simulink model "Linearization2"  (R2022a)
settings: Solver=VariableStepAuto  StartTime=0.0  StopTime=10.0  RelTol=1e-3
undefined symbols (not defined in the file): Aactuator, ac, AeroCoeff, ControlAllocation, DUmax, DUmin, EngineTable, F, fcs, ft, g, hground, IC, kg, LandingGear, Light, LPmethod, m, MIL, Mode_deflection_aileron, Mode_deflection_elevator, Mode_deflection_rudder, Mode_deflection_TVC_y, Mode_deflection_TVC_z, N, Ninv_2nozzle, Ninv_no_nozzle, PIController, s, Sensor, slug, state0, sysID_DAQ, sysID_OBES, Umax_2nozzle, Umax_no_nozzle, Umin_2nozzle, Umin_no_nozzle, WMM2020
libraries: aerolibconvert2 x19, slpidlib x6, simulink x6, sharedutil x4, aerolibatmos2 x3, aerolibwind2 x3, aerolibbdyn x3, aerolibgravity2 x2, sharedtransform x1
(part 1 of 9)
settings Model: Creator=user  LastModifiedBy=user
settings DataIOCC: ExternalInput=getinputstruct(op_trim1)  InitialState=getstatestruct(op_trim1)

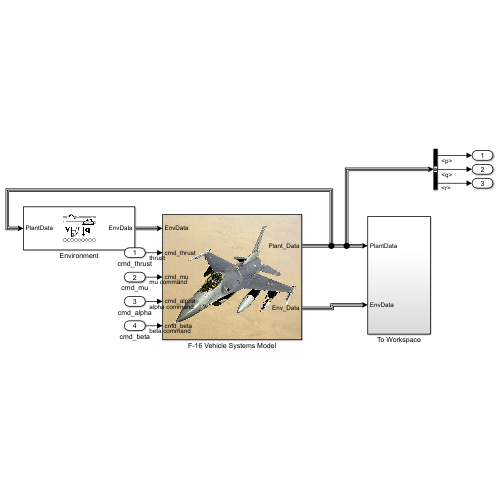
[thumbnail: Simulink's stored preview of the top-level diagram]
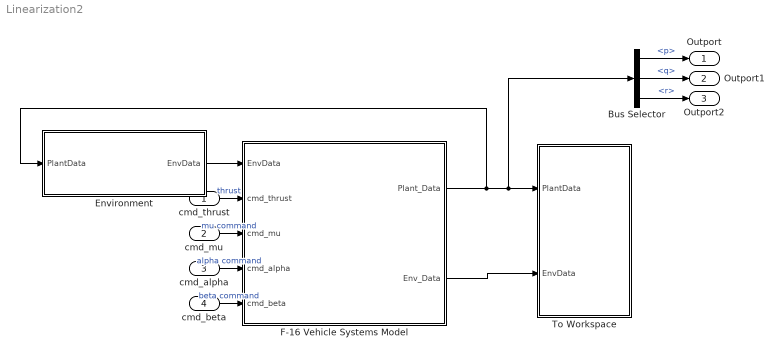
== system Linearization2 ==
  cmd_thrust : Inport
  cmd_mu : Inport  Port=2
  cmd_alpha : Inport  Port=3
  cmd_beta : Inport  Port=4
  Bus Selector : BusSelector  OutputSignals=p,q,r
  Environment : Subsystem
      mask Display:
      | image('aeroenvironment.bmp','center')
      | % 左側 "Icon transparency" 欄位已選擇 "Opaque with ports"，所以埠名稱會自動顯示，不用再宣告
      | % port_label('input',1,'PlantData')
      | % port_label('output',1,'EnvData')
  F-16 Vehicle Systems Model : Subsystem
      mask Display:
      | proj = currentProject;   % 返回一個專案物件proj 代表當前打開的Project專案
      | filepath = fullfile(proj.RootFolder,'\image\F-16_wikipedia.jpg');
      | image(filepath,'center');
      | % 左側 "Icon transparency" 欄位已選擇 "Opaque with ports"，所以埠名稱會自動顯示，不用再宣告
      | % port_label('input',1,'EnvData')
      | % port_label('output',1,'Plant_Data')
      | % port_label('output',2,'Env_Data')
  To Workspace : Subsystem
  Outport : Outport
  Outport1 : Outport  Port=2
  Outport2 : Outport  Port=3
  wires:
  F-16 Vehicle Systems Model/1(Plant_Data) -> Environment/1(PlantData), Bus Selector/1, To Workspace/1(PlantData)
  F-16 Vehicle Systems Model/2(Env_Data) -> To Workspace/2(EnvData)
  Environment/1(EnvData) -> F-16 Vehicle Systems Model/1(EnvData)
  cmd_thrust/1 -> F-16 Vehicle Systems Model/2(cmd_thrust)  "thrust"
  cmd_mu/1 -> F-16 Vehicle Systems Model/3(cmd_mu)  "mu command"
  cmd_alpha/1 -> F-16 Vehicle Systems Model/4(cmd_alpha)  "alpha command"
  cmd_beta/1 -> F-16 Vehicle Systems Model/5(cmd_beta)  "beta command"
  Bus Selector/1 -> Outport/1  "<p>"
  Bus Selector/2 -> Outport1/1  "<q>"
  Bus Selector/3 -> Outport2/1  "<r>"

== system Linearization2/Environment ==
  note: p, q, r
  note: u, v, w
  note: Wind Models
  note: Atmosphere Model
  note: Altitude must be less than 20000 m (approximately 65620 feet).
  note: 建模注意： EnvData Bus 內要指定公制/英制單位
  note: Magnetic Field
  note: Gravity Model
  note: TODO: 改用這個現成模塊...
      | 但NDI控制器內的重力g是用常數，將產生誤差...
  note: TODO: 改用這個現成模塊...
      | 參考MATLAB Help範例 Quadcopter Project
  note: TODO: 改用現成模塊，改成英制。
      | NDI控制器，不會產生誤差，因為可轉成C程式碼
  note: TODO: 參考MATLAB Help範例 HL-20
      | 將風速效應加到氣動力攻角、側滑角、qbar、Mach、V
  In Bus Element1 : Inport  PortName=PlantData  Element=altitude
  In Bus Element2 : Inport  PortName=PlantData  Element=altitude
  In Bus Element3 : Inport  PortName=PlantData  Element=Vt
  In Bus Element4 : Inport  PortName=PlantData  Element=Vt
  In Bus Element5 : Inport  PortName=PlantData  Element=Vt
  In Bus Element : Inport  PortName=PlantData  Element=DCM_be
  COESA Atmosphere Model : aerolibatmos2/COESA Atmosphere Model  Commented=on  units=English (Velocity in ft/s)  spec=1976 COESA-extended U.S. Standard Atmosphere  model=Profile  profile_var=High temperature  profile_percent=1%  profile_alt=5 km (16404 ft)  envelope_var=High temperature  envelope_percent=1%  action=Warning
  Density Conversion : aerolibconvert2/Density Conversion  IU=kg/m^3  OU=slug/ft^3
      settings: SourceProductBaseCode=AE
  Discrete Wind Gust Model : aerolibwind2/Discrete Wind Gust Model  Commented=on  units=English (Velocity in ft/s)  Gx=on  Gy=on  Gz=on  t_0=5  d_m=[120 120 80]  v_m=[3.5 3.5 3.0]
  Dryden Wind Turbulence Model (Continuous (+q +r)) : aerolibwind2/Dryden Wind Turbulence Model  (Continuous (+q -r))  Commented=on  units=English (Velocity in ft/s)  spec=MIL-F-8785C  model=Continuous Dryden (+q +r)  W20=15  Wdeg=0  TurbProb=10^-2 - Light  L_high=533.4  Wingspan=10  ts=0.1  Seed=[23341 23342 23343 23344]  T_on=on
  Dynamic Pressure : Subsystem
  Geoid Height : aerolibgravity2/Geoid Height  Commented=on  units=English  gtype=EGM96  datafile='geoidegm96grid'  dtype=double  action=Warning
      settings: AttributesFormatString=EGM2008 Geoid Data Unavailable  SourceProductBaseCode=AE
  ISA Atmosphere Model : aerolibatmos2/ISA Atmosphere Model  Commented=on  custom=off  g=9.80665  gamma=1.4  R=287.0531  L=0.0065  h_trop=11000  h_strat=20000  rho0=1.225  P0=101325  T0=288.15  h0=0
  "ISP " : Subsystem
  Length Conversion : aerolibconvert2/Length Conversion  IU=ft  OU=m
  Mach Number : Subsystem
  Magnetic Field : Constant  Value=[0 0 0]
  Manual Switch : ManualSwitch
  Manual Switch1 : ManualSwitch  CurrentSetting=0
  Pressure Altitude : aerolibatmos2/Pressure Altitude  Commented=on  units=English  action=Warning
      settings: SourceProductBaseCode=AE
  Sum : Sum  Commented=on  Inputs=+++
  Velocity Conversion : aerolibconvert2/Velocity Conversion  IU=m/s  OU=ft/s
  "WGS84 Gravity Model  " : GravityWGS84  Commented=on  units=English
  Wind Shear Model : aerolibwind2/Wind Shear Model  Commented=on  units=English (Velocity in ft/s)  phase=Category C - Terminal Flight Phase  W_20=15  Wdeg=0
  World Magnetic Model : aerolibgravity2/World Magnetic Model  Commented=on  model=WMM2020 (2020-2025)  customFile='WMM2020.COF'  units=English  time_in=on  month=January  day=1  year=2020  action=Error  h_out=off  dec_out=off  inc_out=off  ti_out=off
      settings: SourceProductBaseCode=AE
  gravity (ft/s^2) : Constant  Value=g
  hground (ft) : Constant  Value=hground
  no wind : Constant  Value=[0 0 0]
  no wind1 : Constant  Value=[0 0 0]
  r2d1 : Gain  Commented=on  Gain=-1  SaturateOnIntegerOverflow=on  OutDataTypeStr=Inherit: Same as input  ParamDataTypeStr=Inherit: Same as input
  r2d2 : Gain  Gain=-1  SaturateOnIntegerOverflow=on  OutDataTypeStr=Inherit: Same as input  ParamDataTypeStr=Inherit: Same as input
  Out Bus Element : Outport  PortName=EnvData  Element=Pressure
  Out Bus Element1 : Outport  PortName=EnvData  Element=AirDensity
  Out Bus Element2 : Outport  PortName=EnvData  Element=qbar
  Out Bus Element3 : Outport  PortName=EnvData  Element=Mach
  Out Bus Element4 : Outport  PortName=EnvData  Element=g
  Out Bus Element5 : Outport  PortName=EnvData  Element=hground
  Out Bus Element6 : Outport  PortName=EnvData  Element=MagneticField_NED
  Out Bus Element7 : Outport  PortName=EnvData  Element=AirTemperature_K
  Out Bus Element8 : Outport  PortName=EnvData  Element=SoundSpeed_ms
  Out Bus Element9 : Outport  PortName=EnvData  Element=WindVelocity
  Out Bus Element10 : Outport  PortName=EnvData  Element=WindAngularRates
  wires:
  "ISP "/1(T (K)) -> Out Bus Element7/1
  "ISP "/3(P (HPa)) -> Out Bus Element/1
  "ISP "/4(rho (kg/m^3)) -> Density Conversion/1, Out Bus Element1/1
  hground (ft)/1 -> Out Bus Element5/1
  gravity (ft/s^2)/1 -> Out Bus Element4/1  "Gravity_NED"
  Magnetic Field/1 -> Out Bus Element6/1  "MagneticField_NED"
  In Bus Element1/1 -> r2d2/1
  r2d2/1 -> Length Conversion/1  "h(ft)"
  Length Conversion/1 -> "ISP "/1(h(m))
  "ISP "/2(a (m/s)) -> Out Bus Element8/1, Velocity Conversion/1
  Mach Number/1(Mach) -> Out Bus Element3/1
  Dynamic Pressure/1(qbar) -> Out Bus Element2/1
  Density Conversion/1 -> Dynamic Pressure/2(rho)
  In Bus Element3/1 -> Dynamic Pressure/1(Vt)  "Vt (ft/s)"
  In Bus Element4/1 -> Mach Number/1(Vt)  "Vt (ft/s)"
  Velocity Conversion/1 -> Mach Number/2(a)
  COESA Atmosphere Model/3 -> Pressure Altitude/1
  r2d1/1 -> Dryden Wind Turbulence Model (Continuous (+q +r))/1, Wind Shear Model/1  "h(ft)"
  In Bus Element2/1 -> r2d1/1
  In Bus Element5/1 -> Dryden Wind Turbulence Model (Continuous (+q +r))/2, Discrete Wind Gust Model/1  "Vt (ft/s)"
  In Bus Element/1 -> Wind Shear Model/2, Dryden Wind Turbulence Model (Continuous (+q +r))/3
  Dryden Wind Turbulence Model (Continuous (+q +r))/1 -> Sum/2
  Discrete Wind Gust Model/1 -> Sum/3
  Wind Shear Model/1 -> Sum/1
  Dryden Wind Turbulence Model (Continuous (+q +r))/2 -> Manual Switch1/1  "WindAngularRates"
  Sum/1 -> Manual Switch/2  "WindVelocity"
  Manual Switch/1 -> Out Bus Element9/1
  no wind/1 -> Manual Switch/1
  Manual Switch1/1 -> Out Bus Element10/1
  no wind1/1 -> Manual Switch1/2

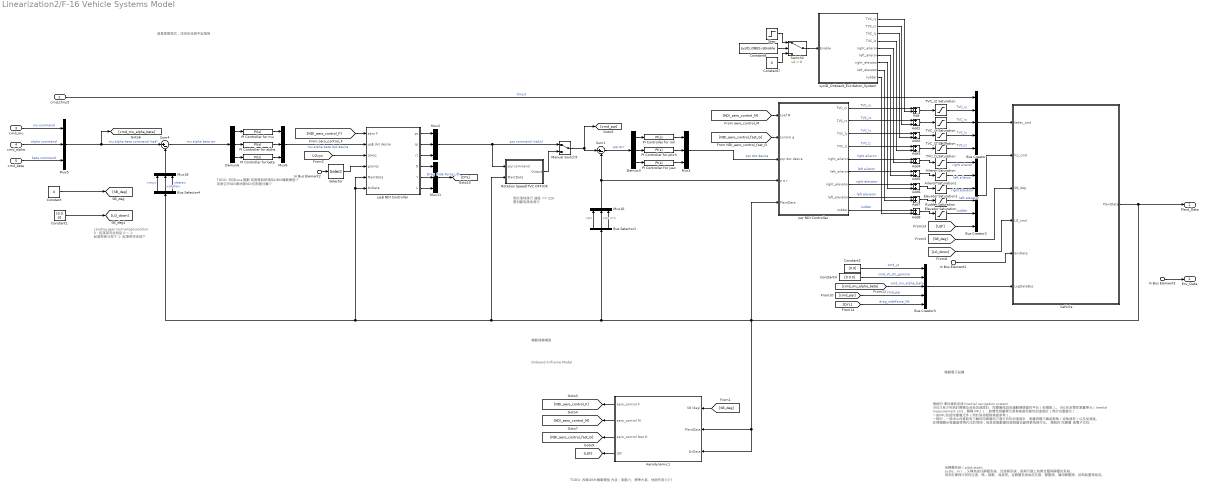
== system Linearization2/F-16 Vehicle Systems Model ==
  note: 機載飛機模型
  note: Onboard Airframe Model
  note: TODO: 改成local變數
      | 或者應該新增為OBM機載模型!?
      | 或者空中NDI跟地面NDI控制器分離!?
  note: 用於落地滑行
      | 速度 <= 220 會判斷為落地滑行
  note: 這是家維程式，改成包含庭宇起落架
  note: 機載電子設備
  note: 全靜壓系統（pitot-static system），又稱為皮托靜壓系統、空速管系統，是飛行器上收集全壓與靜壓的系統，
      | 用來計算飛行時的空速、馬赫數、海拔等。全靜壓系統由皮托管、靜壓源、備用靜壓源、加熱裝置等組成。
  note: 傳統的 慣性導航系統(inertial navigation system (INS))至少包括計算機及含有加速度計、陀螺儀或其他運動傳感器的平台（或模組）。
      | INS包含慣性測量單元（Inertial measurement unit，簡稱 IMU ），該慣性測量單元具有角度和線性加速度計（用於位置變化）；
      | 一些IMU包括陀螺儀元件（用於保持絕對角度參考）。
      | 一般的，一個IMU內會裝有三軸的陀螺儀和三個方向的加速度計，測量物體三軸姿態角（或角速率）以及加速度。
      |
      | 在飛機顯示裝置變得現代化的同時，為其採集數據的感測器也變得更為現代化。
      | 傳統的 陀螺儀 被電子式的 航向姿態基準系統 （AHRS）與 大氣數據計算機 （ADC）所取代，
      | 在增加可靠性的同時也降低了成本、簡化了維護。
      | 此外， GPS 接收器也被整合進了玻璃駕駛艙之中。
  note: Landing gear normalized position
      | 0 : 起落架完全收起
      | 0 ~ 1: 起落架部分放下
      | 1: 起落架完全放下
  note: TODO: 改稱OBM機載模型
      | 內含：氣動力、標準大氣、地面作用力(?)
  In Bus Element1 : Inport  PortName=EnvData
  In Bus Element3 : Inport  PortName=EnvData
  In Bus Element2 : Inport  PortName=EnvData  Element=g
  cmd_thrust : Inport  Port=2
  cmd_mu : Inport  Port=3
  cmd_alpha : Inport  Port=4
  cmd_beta : Inport  Port=5
  Add{,1..8} (9 alike) : Sum
  Aerodynamic1 : Subsystem
  Aileron Saturation : Saturate  UpperLimit=Aactuator.aileron.AngleLimitUpper  LowerLimit=Aactuator.aileron.AngleLimitLower
  Aileron Saturation1 : Saturate  UpperLimit=Aactuator.aileron.AngleLimitUpper  LowerLimit=Aactuator.aileron.AngleLimitLower
  Bus Creator : BusCreator  Inputs=5
  Bus Creator2 : BusCreator  Inputs=6
  Bus Creator3 : BusCreator  Inputs=5
  Bus Selector1 : BusSelector  OutputSignals=p,q,r
  Bus Selector4 : BusSelector  OutputSignals=mu,alpha,beta
  Constant : Constant  Value=0
  Constant1 : Constant  Value=[0 0 0]
  Constant2 : Constant  Value=[0 0]
  Constant4 : Constant  Value=[0 0 0]
  Constant7 : Constant  Value=0
  Constant8 : Constant  Value=sysID_OBES.isEnable
  Demux3 : Demux  Outputs=3
  Demux6 : Demux  Outputs=3
  Elevator Saturation : Saturate  UpperLimit=Aactuator.elevator.AngleLimitUpper  LowerLimit=Aactuator.elevator.AngleLimitLower
  Elevator Saturation1 : Saturate  UpperLimit=Aactuator.elevator.AngleLimitUpper  LowerLimit=Aactuator.elevator.AngleLimitLower
  Manual Switch5 : ManualSwitch
  Mux{1..2,5..6,11,16,18} (7 alike) : Mux  Inputs=3
  PI Controller for alpha : slpidlib/PID Controller  Controller=PI  Form=Parallel  TimeDomain=Continuous-time  UseExternalTs=off  SampleTime=-1  IntegratorMethod=Forward Euler  FilterMethod=Forward Euler  ControllerParametersSource=internal  P=PIController.alpha.P  I=PIController.alpha.I  UseKiTs=off  D=0  N=100  UseFilter=on  TunerSelectOption=Transfer Function Based (PID Tuner App)  InitialConditionSource=internal  InitialConditionForIntegrator=0  InitialConditionForFilter=0  DifferentiatorICPrevScaledInput=0  ExternalReset=none  TrackingMode=off  Kt=1  LimitOutput=off  SatLimitsSource=internal  UpperSaturationLimit=inf  LowerSaturationLimit=-inf  LinearizeAsGain=on  AntiWindupMode=none  Kb=1  POutMin=[]  POutMax=[]  IOutMin=[]  IOutMax=[]  DOutMin=[]  DOutMax=[]  NOutMin=[]  NOutMax=[]  SumOutMin=[]  SumOutMax=[]  SaturationOutMin=[]  SaturationOutMax=[]  PParamMin=[]  PParamMax=[]  IParamMin=[]  IParamMax=[]  DParamMin=[]  DParamMax=[]  NParamMin=[]  NParamMax=[]  KbParamMin=[]  KbParamMax=[]  KtParamMin=[]  KtParamMax=[]  KbOutMin=[]  KbOutMax=[]  KtOutMin=[]  KtOutMax=[]  IntegratorOutMin=[]  IntegratorOutMax=[]  FilterOutMin=[]  FilterOutMax=[]  SumI1OutMin=[]  SumI1OutMax=[]  SumI2OutMin=[]  SumI2OutMax=[]  SumI3OutMin=[]  SumI3OutMax=[]  SumI4OutMin=[]  SumI4OutMax=[]  SumDOutMin=[]  SumDOutMax=[]  DifferentiatorOutMin=[]  DifferentiatorOutMax=[]  FilterDiffOutCoefMin=[]  FilterDiffOutCoefMax=[]  ReciprocalOutMin=[]  ReciprocalOutMax=[]  SumDenOutMin=[]  SumDenOutMax=[]  SumNumOutMin=[]  SumNumOutMax=[]  DivideOutMin=[]  DivideOutMax=[]  UdiffTsProdOutMin=[]  UdiffTsProdOutMax=[]  NTsProdOutMin=[]  NTsProdOutMax=[]  UintegralTsProdOutMin=[]  UintegralTsProdOutMax=[]  UngainTsProdOutMin=[]  UngainTsProdOutMax=[]  IntegratorContinuousStateAttributes=''  IntegratorStateMustResolveToSignalObject=off  IntegratorRTWStateStorageClass=Auto  FilterContinuousStateAttributes=''  FilterStateMustResolveToSignalObject=off  FilterRTWStateStorageClass=Auto  ParallelPVariant=InternalParameters  IdealPVariant=Disabled  IVariant=InternalParameters  DVariant=Disabled  IntegratorVariant=Continuous  SatVariant=Disabled  AWVariant=Passthrough  PCopyVariant=Disabled  TRVariant=Disabled  FdbkBlocksVariant=Forward  IdealPFdbkVariant=Disabled  SatFdbkVariant=Disabled  DerivativeFilterVariant=Disabled  NVariant=Disabled  NCopyVariant=Disabled_SignalSpec  FilterICVariant=Disabled  IntegratorICVariant=InternalICs  ExternalResetVariant=Disabled  TRSumVariant=Passthrough  SumFdbkVariant=Disabled  SumVariant=Sum_PI  TsampFilterVariant=InternalTs  TsampNgainVariant=Passthrough  TsampIntegralVariant=Passthrough  ExternalSaturationOutDataTypeStr=Inherit: Same as second input  aMode=0
  PI Controller for beta : slpidlib/PID Controller  Controller=PI  Form=Parallel  TimeDomain=Continuous-time  UseExternalTs=off  SampleTime=-1  IntegratorMethod=Forward Euler  FilterMethod=Forward Euler  ControllerParametersSource=internal  P=PIController.beta.P  I=PIController.beta.I  UseKiTs=off  D=0  N=100  UseFilter=on  TunerSelectOption=Transfer Function Based (PID Tuner App)  InitialConditionSource=internal  InitialConditionForIntegrator=0  InitialConditionForFilter=0  DifferentiatorICPrevScaledInput=0  ExternalReset=none  TrackingMode=off  Kt=1  LimitOutput=off  SatLimitsSource=internal  UpperSaturationLimit=inf  LowerSaturationLimit=-inf  LinearizeAsGain=on  AntiWindupMode=none  Kb=1  POutMin=[]  POutMax=[]  IOutMin=[]  IOutMax=[]  DOutMin=[]  DOutMax=[]  NOutMin=[]  NOutMax=[]  SumOutMin=[]  SumOutMax=[]  SaturationOutMin=[]  SaturationOutMax=[]  PParamMin=[]  PParamMax=[]  IParamMin=[]  IParamMax=[]  DParamMin=[]  DParamMax=[]  NParamMin=[]  NParamMax=[]  KbParamMin=[]  KbParamMax=[]  KtParamMin=[]  KtParamMax=[]  KbOutMin=[]  KbOutMax=[]  KtOutMin=[]  KtOutMax=[]  IntegratorOutMin=[]  IntegratorOutMax=[]  FilterOutMin=[]  FilterOutMax=[]  SumI1OutMin=[]  SumI1OutMax=[]  SumI2OutMin=[]  SumI2OutMax=[]  SumI3OutMin=[]  SumI3OutMax=[]  SumI4OutMin=[]  SumI4OutMax=[]  SumDOutMin=[]  SumDOutMax=[]  DifferentiatorOutMin=[]  DifferentiatorOutMax=[]  FilterDiffOutCoefMin=[]  FilterDiffOutCoefMax=[]  ReciprocalOutMin=[]  ReciprocalOutMax=[]  SumDenOutMin=[]  SumDenOutMax=[]  SumNumOutMin=[]  SumNumOutMax=[]  DivideOutMin=[]  DivideOutMax=[]  UdiffTsProdOutMin=[]  UdiffTsProdOutMax=[]  NTsProdOutMin=[]  NTsProdOutMax=[]  UintegralTsProdOutMin=[]  UintegralTsProdOutMax=[]  UngainTsProdOutMin=[]  UngainTsProdOutMax=[]  IntegratorContinuousStateAttributes=''  IntegratorStateMustResolveToSignalObject=off  IntegratorRTWStateStorageClass=Auto  FilterContinuousStateAttributes=''  FilterStateMustResolveToSignalObject=off  FilterRTWStateStorageClass=Auto  ParallelPVariant=InternalParameters  IdealPVariant=Disabled  IVariant=InternalParameters  DVariant=Disabled  IntegratorVariant=Continuous  SatVariant=Disabled  AWVariant=Passthrough  PCopyVariant=Disabled  TRVariant=Disabled  FdbkBlocksVariant=Forward  IdealPFdbkVariant=Disabled  SatFdbkVariant=Disabled  DerivativeFilterVariant=Disabled  NVariant=Disabled  NCopyVariant=Disabled_SignalSpec  FilterICVariant=Disabled  IntegratorICVariant=InternalICs  ExternalResetVariant=Disabled  TRSumVariant=Passthrough  SumFdbkVariant=Disabled  SumVariant=Sum_PI  TsampFilterVariant=InternalTs  TsampNgainVariant=Passthrough  TsampIntegralVariant=Passthrough  ExternalSaturationOutDataTypeStr=Inherit: Same as second input  aMode=0
  PI Controller for mu : slpidlib/PID Controller  Controller=PI  Form=Parallel  TimeDomain=Continuous-time  UseExternalTs=off  SampleTime=-1  IntegratorMethod=Forward Euler  FilterMethod=Forward Euler  ControllerParametersSource=internal  P=PIController.mu.P  I=PIController.mu.I  UseKiTs=off  D=0  N=100  UseFilter=on  TunerSelectOption=Transfer Function Based (PID Tuner App)  InitialConditionSource=internal  InitialConditionForIntegrator=0  InitialConditionForFilter=0  DifferentiatorICPrevScaledInput=0  ExternalReset=none  TrackingMode=off  Kt=1  LimitOutput=off  SatLimitsSource=internal  UpperSaturationLimit=inf  LowerSaturationLimit=-inf  LinearizeAsGain=on  AntiWindupMode=none  Kb=1  POutMin=[]  POutMax=[]  IOutMin=[]  IOutMax=[]  DOutMin=[]  DOutMax=[]  NOutMin=[]  NOutMax=[]  SumOutMin=[]  SumOutMax=[]  SaturationOutMin=[]  SaturationOutMax=[]  PParamMin=[]  PParamMax=[]  IParamMin=[]  IParamMax=[]  DParamMin=[]  DParamMax=[]  NParamMin=[]  NParamMax=[]  KbParamMin=[]  KbParamMax=[]  KtParamMin=[]  KtParamMax=[]  KbOutMin=[]  KbOutMax=[]  KtOutMin=[]  KtOutMax=[]  IntegratorOutMin=[]  IntegratorOutMax=[]  FilterOutMin=[]  FilterOutMax=[]  SumI1OutMin=[]  SumI1OutMax=[]  SumI2OutMin=[]  SumI2OutMax=[]  SumI3OutMin=[]  SumI3OutMax=[]  SumI4OutMin=[]  SumI4OutMax=[]  SumDOutMin=[]  SumDOutMax=[]  DifferentiatorOutMin=[]  DifferentiatorOutMax=[]  FilterDiffOutCoefMin=[]  FilterDiffOutCoefMax=[]  ReciprocalOutMin=[]  ReciprocalOutMax=[]  SumDenOutMin=[]  SumDenOutMax=[]  SumNumOutMin=[]  SumNumOutMax=[]  DivideOutMin=[]  DivideOutMax=[]  UdiffTsProdOutMin=[]  UdiffTsProdOutMax=[]  NTsProdOutMin=[]  NTsProdOutMax=[]  UintegralTsProdOutMin=[]  UintegralTsProdOutMax=[]  UngainTsProdOutMin=[]  UngainTsProdOutMax=[]  IntegratorContinuousStateAttributes=''  IntegratorStateMustResolveToSignalObject=off  IntegratorRTWStateStorageClass=Auto  FilterContinuousStateAttributes=''  FilterStateMustResolveToSignalObject=off  FilterRTWStateStorageClass=Auto  ParallelPVariant=InternalParameters  IdealPVariant=Disabled  IVariant=InternalParameters  DVariant=Disabled  IntegratorVariant=Continuous  SatVariant=Disabled  AWVariant=Passthrough  PCopyVariant=Disabled  TRVariant=Disabled  FdbkBlocksVariant=Forward  IdealPFdbkVariant=Disabled  SatFdbkVariant=Disabled  DerivativeFilterVariant=Disabled  NVariant=Disabled  NCopyVariant=Disabled_SignalSpec  FilterICVariant=Disabled  IntegratorICVariant=InternalICs  ExternalResetVariant=Disabled  TRSumVariant=Passthrough  SumFdbkVariant=Disabled  SumVariant=Sum_PI  TsampFilterVariant=InternalTs  TsampNgainVariant=Passthrough  TsampIntegralVariant=Passthrough  ExternalSaturationOutDataTypeStr=Inherit: Same as second input  aMode=0
  PI Controller for pitch : slpidlib/PID Controller  Controller=PI  Form=Parallel  TimeDomain=Continuous-time  UseExternalTs=off  SampleTime=-1  IntegratorMethod=Forward Euler  FilterMethod=Forward Euler  ControllerParametersSource=internal  P=PIController.q.P  I=PIController.q.I  UseKiTs=off  D=0  N=100  UseFilter=on  TunerSelectOption=Transfer Function Based (PID Tuner App)  InitialConditionSource=internal  InitialConditionForIntegrator=0  InitialConditionForFilter=0  DifferentiatorICPrevScaledInput=0  ExternalReset=none  TrackingMode=off  Kt=1  LimitOutput=off  SatLimitsSource=internal  UpperSaturationLimit=inf  LowerSaturationLimit=-inf  LinearizeAsGain=on  AntiWindupMode=none  Kb=1  POutMin=[]  POutMax=[]  IOutMin=[]  IOutMax=[]  DOutMin=[]  DOutMax=[]  NOutMin=[]  NOutMax=[]  SumOutMin=[]  SumOutMax=[]  SaturationOutMin=[]  SaturationOutMax=[]  PParamMin=[]  PParamMax=[]  IParamMin=[]  IParamMax=[]  DParamMin=[]  DParamMax=[]  NParamMin=[]  NParamMax=[]  KbParamMin=[]  KbParamMax=[]  KtParamMin=[]  KtParamMax=[]  KbOutMin=[]  KbOutMax=[]  KtOutMin=[]  KtOutMax=[]  IntegratorOutMin=[]  IntegratorOutMax=[]  FilterOutMin=[]  FilterOutMax=[]  SumI1OutMin=[]  SumI1OutMax=[]  SumI2OutMin=[]  SumI2OutMax=[]  SumI3OutMin=[]  SumI3OutMax=[]  SumI4OutMin=[]  SumI4OutMax=[]  SumDOutMin=[]  SumDOutMax=[]  DifferentiatorOutMin=[]  DifferentiatorOutMax=[]  FilterDiffOutCoefMin=[]  FilterDiffOutCoefMax=[]  ReciprocalOutMin=[]  ReciprocalOutMax=[]  SumDenOutMin=[]  SumDenOutMax=[]  SumNumOutMin=[]  SumNumOutMax=[]  DivideOutMin=[]  DivideOutMax=[]  UdiffTsProdOutMin=[]  UdiffTsProdOutMax=[]  NTsProdOutMin=[]  NTsProdOutMax=[]  UintegralTsProdOutMin=[]  UintegralTsProdOutMax=[]  UngainTsProdOutMin=[]  UngainTsProdOutMax=[]  IntegratorContinuousStateAttributes=''  IntegratorStateMustResolveToSignalObject=off  IntegratorRTWStateStorageClass=Auto  FilterContinuousStateAttributes=''  FilterStateMustResolveToSignalObject=off  FilterRTWStateStorageClass=Auto  ParallelPVariant=InternalParameters  IdealPVariant=Disabled  IVariant=InternalParameters  DVariant=Disabled  IntegratorVariant=Continuous  SatVariant=Disabled  AWVariant=Passthrough  PCopyVariant=Disabled  TRVariant=Disabled  FdbkBlocksVariant=Forward  IdealPFdbkVariant=Disabled  SatFdbkVariant=Disabled  DerivativeFilterVariant=Disabled  NVariant=Disabled  NCopyVariant=Disabled_SignalSpec  FilterICVariant=Disabled  IntegratorICVariant=InternalICs  ExternalResetVariant=Disabled  TRSumVariant=Passthrough  SumFdbkVariant=Disabled  SumVariant=Sum_PI  TsampFilterVariant=InternalTs  TsampNgainVariant=Passthrough  TsampIntegralVariant=Passthrough  ExternalSaturationOutDataTypeStr=Inherit: Same as second input  aMode=0
  PI Controller for roll : slpidlib/PID Controller  Controller=PI  Form=Parallel  TimeDomain=Continuous-time  UseExternalTs=off  SampleTime=-1  IntegratorMethod=Forward Euler  FilterMethod=Forward Euler  ControllerParametersSource=internal  P=PIController.p.P  I=PIController.p.I  UseKiTs=off  D=0  N=100  UseFilter=on  TunerSelectOption=Transfer Function Based (PID Tuner App)  InitialConditionSource=internal  InitialConditionForIntegrator=0  InitialConditionForFilter=0  DifferentiatorICPrevScaledInput=0  ExternalReset=none  TrackingMode=off  Kt=1  LimitOutput=off  SatLimitsSource=internal  UpperSaturationLimit=inf  LowerSaturationLimit=-inf  LinearizeAsGain=on  AntiWindupMode=none  Kb=1  POutMin=[]  POutMax=[]  IOutMin=[]  IOutMax=[]  DOutMin=[]  DOutMax=[]  NOutMin=[]  NOutMax=[]  SumOutMin=[]  SumOutMax=[]  SaturationOutMin=[]  SaturationOutMax=[]  PParamMin=[]  PParamMax=[]  IParamMin=[]  IParamMax=[]  DParamMin=[]  DParamMax=[]  NParamMin=[]  NParamMax=[]  KbParamMin=[]  KbParamMax=[]  KtParamMin=[]  KtParamMax=[]  KbOutMin=[]  KbOutMax=[]  KtOutMin=[]  KtOutMax=[]  IntegratorOutMin=[]  IntegratorOutMax=[]  FilterOutMin=[]  FilterOutMax=[]  SumI1OutMin=[]  SumI1OutMax=[]  SumI2OutMin=[]  SumI2OutMax=[]  SumI3OutMin=[]  SumI3OutMax=[]  SumI4OutMin=[]  SumI4OutMax=[]  SumDOutMin=[]  SumDOutMax=[]  DifferentiatorOutMin=[]  DifferentiatorOutMax=[]  FilterDiffOutCoefMin=[]  FilterDiffOutCoefMax=[]  ReciprocalOutMin=[]  ReciprocalOutMax=[]  SumDenOutMin=[]  SumDenOutMax=[]  SumNumOutMin=[]  SumNumOutMax=[]  DivideOutMin=[]  DivideOutMax=[]  UdiffTsProdOutMin=[]  UdiffTsProdOutMax=[]  NTsProdOutMin=[]  NTsProdOutMax=[]  UintegralTsProdOutMin=[]  UintegralTsProdOutMax=[]  UngainTsProdOutMin=[]  UngainTsProdOutMax=[]  IntegratorContinuousStateAttributes=''  IntegratorStateMustResolveToSignalObject=off  IntegratorRTWStateStorageClass=Auto  FilterContinuousStateAttributes=''  FilterStateMustResolveToSignalObject=off  FilterRTWStateStorageClass=Auto  ParallelPVariant=InternalParameters  IdealPVariant=Disabled  IVariant=InternalParameters  DVariant=Disabled  IntegratorVariant=Continuous  SatVariant=Disabled  AWVariant=Passthrough  PCopyVariant=Disabled  TRVariant=Disabled  FdbkBlocksVariant=Forward  IdealPFdbkVariant=Disabled  SatFdbkVariant=Disabled  DerivativeFilterVariant=Disabled  NVariant=Disabled  NCopyVariant=Disabled_SignalSpec  FilterICVariant=Disabled  IntegratorICVariant=InternalICs  ExternalResetVariant=Disabled  TRSumVariant=Passthrough  SumFdbkVariant=Disabled  SumVariant=Sum_PI  TsampFilterVariant=InternalTs  TsampNgainVariant=Passthrough  TsampIntegralVariant=Passthrough  ExternalSaturationOutDataTypeStr=Inherit: Same as second input  aMode=0
  PI Controller for yaw : slpidlib/PID Controller  Controller=PI  Form=Parallel  TimeDomain=Continuous-time  UseExternalTs=off  SampleTime=-1  IntegratorMethod=Forward Euler  FilterMethod=Forward Euler  ControllerParametersSource=internal  P=PIController.r.P  I=PIController.r.I  UseKiTs=off  D=0  N=100  UseFilter=on  TunerSelectOption=Transfer Function Based (PID Tuner App)  InitialConditionSource=internal  InitialConditionForIntegrator=0  InitialConditionForFilter=0  DifferentiatorICPrevScaledInput=0  ExternalReset=none  TrackingMode=off  Kt=1  LimitOutput=off  SatLimitsSource=internal  UpperSaturationLimit=inf  LowerSaturationLimit=-inf  LinearizeAsGain=on  AntiWindupMode=none  Kb=1  POutMin=[]  POutMax=[]  IOutMin=[]  IOutMax=[]  DOutMin=[]  DOutMax=[]  NOutMin=[]  NOutMax=[]  SumOutMin=[]  SumOutMax=[]  SaturationOutMin=[]  SaturationOutMax=[]  PParamMin=[]  PParamMax=[]  IParamMin=[]  IParamMax=[]  DParamMin=[]  DParamMax=[]  NParamMin=[]  NParamMax=[]  KbParamMin=[]  KbParamMax=[]  KtParamMin=[]  KtParamMax=[]  KbOutMin=[]  KbOutMax=[]  KtOutMin=[]  KtOutMax=[]  IntegratorOutMin=[]  IntegratorOutMax=[]  FilterOutMin=[]  FilterOutMax=[]  SumI1OutMin=[]  SumI1OutMax=[]  SumI2OutMin=[]  SumI2OutMax=[]  SumI3OutMin=[]  SumI3OutMax=[]  SumI4OutMin=[]  SumI4OutMax=[]  SumDOutMin=[]  SumDOutMax=[]  DifferentiatorOutMin=[]  DifferentiatorOutMax=[]  FilterDiffOutCoefMin=[]  FilterDiffOutCoefMax=[]  ReciprocalOutMin=[]  ReciprocalOutMax=[]  SumDenOutMin=[]  SumDenOutMax=[]  SumNumOutMin=[]  SumNumOutMax=[]  DivideOutMin=[]  DivideOutMax=[]  UdiffTsProdOutMin=[]  UdiffTsProdOutMax=[]  NTsProdOutMin=[]  NTsProdOutMax=[]  UintegralTsProdOutMin=[]  UintegralTsProdOutMax=[]  UngainTsProdOutMin=[]  UngainTsProdOutMax=[]  IntegratorContinuousStateAttributes=''  IntegratorStateMustResolveToSignalObject=off  IntegratorRTWStateStorageClass=Auto  FilterContinuousStateAttributes=''  FilterStateMustResolveToSignalObject=off  FilterRTWStateStorageClass=Auto  ParallelPVariant=InternalParameters  IdealPVariant=Disabled  IVariant=InternalParameters  DVariant=Disabled  IntegratorVariant=Continuous  SatVariant=Disabled  AWVariant=Passthrough  PCopyVariant=Disabled  TRVariant=Disabled  FdbkBlocksVariant=Forward  IdealPFdbkVariant=Disabled  SatFdbkVariant=Disabled  DerivativeFilterVariant=Disabled  NVariant=Disabled  NCopyVariant=Disabled_SignalSpec  FilterICVariant=Disabled  IntegratorICVariant=InternalICs  ExternalResetVariant=Disabled  TRSumVariant=Passthrough  SumFdbkVariant=Disabled  SumVariant=Sum_PI  TsampFilterVariant=InternalTs  TsampNgainVariant=Passthrough  TsampIntegralVariant=Passthrough  ExternalSaturationOutDataTypeStr=Inherit: Same as second input  aMode=0
  Rotation Speed(TVC OFF)OK : Subsystem
  Rudder Saturation : Saturate  UpperLimit=Aactuator.rudder.AngleLimitUpper  LowerLimit=Aactuator.rudder.AngleLimitLower
  Selector : Selector  InputPortWidth=3  IndexOptions=Index vector (dialog)  Indices=3  OutputSizes=1
  Step : Step  Time=sysID_OBES.start_time  SampleTime=0
  Sum1 : Sum  Inputs=|+-
  Sum4 : Sum  Inputs=|+-
  Switch2 : Switch  Criteria=u2 > Threshold  SaturateOnIntegerOverflow=off  InputSameDT=off
  TVC_lY Saturation : Saturate  UpperLimit=Aactuator.TVC_Z.AngleLimitUpper  LowerLimit=Aactuator.TVC_Z.AngleLimitLower
  TVC_lZ Saturation : Saturate  UpperLimit=Aactuator.TVC_Y.AngleLimitUpper  LowerLimit=Aactuator.TVC_Y.AngleLimitLower
  TVC_rY Saturation : Saturate  UpperLimit=Aactuator.TVC_Z.AngleLimitUpper  LowerLimit=Aactuator.TVC_Z.AngleLimitLower
  TVC_rZ Saturation : Saturate  UpperLimit=Aactuator.TVC_Y.AngleLimitUpper  LowerLimit=Aactuator.TVC_Y.AngleLimitLower
  Vehicle : Subsystem
  pqr NDI Controller : Subsystem  VariantControl=TVC ON
  sysID_Onboard_Excitation_System : Subsystem
  μαβ NDI Controller : Subsystem
  Plant_Data : Outport
  Env_Data : Outport  Port=2
  wires:
  Aerodynamic1/3(aero_control fast G) -> [NDI_aero_control_fast_G]
  PI Controller for yaw/1 -> Mux1/3
  Demux3/2 -> PI Controller for pitch/1
  PI Controller for roll/1 -> Mux1/1
  Bus Selector1/2 -> Mux16/2  "<q>"
  Demux3/3 -> PI Controller for yaw/1
  Mux2/1 -> Manual Switch5/1, Rotation Speed(TVC OFF)OK/1(pqr command)  "pqr command (rad/s)"
  Bus Selector1/3 -> Mux16/3  "<r>"
  [SB_deg] -> Aerodynamic1/1(SB (deg))
  Bus Selector1/1 -> Mux16/1  "<p>"
  [SB_deg] -> Vehicle/3(" SB_deg")
  Aerodynamic1/2(aero_control M) -> [NDI_aero_control_M]
  Mux16/1 -> pqr NDI Controller/4(p q r), Sum1/2
  Aerodynamic1/1(aero_control F) -> [NDI_aero_control_F]
  PI Controller for pitch/1 -> Mux1/2
  In Bus Element3/1 -> Env_Data/1
  Demux3/1 -> PI Controller for roll/1
  Sum1/1 -> Demux3/1  "pqr err"
  PI Controller for beta/1 -> Mux6/3
  Mux6/1 -> μαβ NDI Controller/2(μαβ dot desire)  "mu alpha beta dot desire"
  Bus Selector4/3 -> Mux18/3  "<beta>"
  Mux5/1 -> [cmd_mu_alpha_beta], Sum4/1  "mu alpha beta command (rad)"
  Sum4/1 -> Demux6/1  "mu alpha beta err"
  PI Controller for mu/1 -> Mux6/1
  Bus Selector4/1 -> Mux18/1  "<mu>"
  Bus Selector4/2 -> Mux18/2  "<alpha>"
  Mux18/1 -> Sum4/2
  Demux6/1 -> PI Controller for mu/1
  PI Controller for alpha/1 -> Mux6/2
  μαβ NDI Controller/1(pc) -> Mux2/1
  [LGxyz] -> μαβ NDI Controller/3(LGxyz)
  [NDI_aero_control_F] -> μαβ NDI Controller/1(aero F)
  μαβ NDI Controller/5(Y) -> Mux11/2
  μαβ NDI Controller/3(rc) -> Mux2/3
  μαβ NDI Controller/2(qc) -> Mux2/2
  μαβ NDI Controller/4(D) -> Mux11/1
  Demux6/2 -> PI Controller for alpha/1
  Demux6/3 -> PI Controller for beta/1
  Mux11/1 -> [DYL]  "Drag  Side Force Lift"
  μαβ NDI Controller/6(L) -> Mux11/3
  Bus Creator2/1 -> Vehicle/2(fcs_cmd)
  Bus Creator/1 -> Vehicle/1(fadec_cmd)
  cmd_thrust/1 -> Bus Creator/1  "thrust"
  Elevator Saturation1/1 -> Bus Creator2/3  "right elevator"
  Elevator Saturation/1 -> Bus Creator2/4  "left elevator"
  Aileron Saturation1/1 -> Bus Creator2/2  "left aileron"
  Aileron Saturation/1 -> Bus Creator2/1  "right aileron"
  Rudder Saturation/1 -> Bus Creator2/5  "rudder"
  TVC_rZ Saturation/1 -> Bus Creator/2  "TVC_ry"
  TVC_rY Saturation/1 -> Bus Creator/3  "TVC_rz"
  TVC_lZ Saturation/1 -> Bus Creator/4  "TVC_ly"
  TVC_lY Saturation/1 -> Bus Creator/5  "TVC_lz"
  [LG_down] -> Vehicle/4(LG_cmd)
  Rotation Speed(TVC OFF)OK/1(Output) -> Manual Switch5/2
  Constant1/1 -> [LG_down]
  Constant/1 -> [SB_deg]
  In Bus Element2/1 -> Selector/1
  Selector/1 -> μαβ NDI Controller/4(gravity)
  sysID_Onboard_Excitation_System/9(rudder) -> Add8/2
  sysID_Onboard_Excitation_System/8(left_elevator) -> Add7/2
  sysID_Onboard_Excitation_System/7(right_elevator) -> Add6/2
  sysID_Onboard_Excitation_System/6(left_aileron) -> Add5/2
  sysID_Onboard_Excitation_System/5(right_aileron) -> Add4/2
  sysID_Onboard_Excitation_System/4(TVC_lz) -> Add3/2
  sysID_Onboard_Excitation_System/3(TVC_ly) -> Add2/2
  sysID_Onboard_Excitation_System/2(TVC_rz) -> Add1/2
  pqr NDI Controller/9(rudder) -> Add8/1  "rudder"
  sysID_Onboard_Excitation_System/1(TVC_ry) -> Add/2
  pqr NDI Controller/4("TVC_lz ") -> Add3/1  "TVC_lz"
  pqr NDI Controller/3("TVC_ly ") -> Add2/1  "TVC_ly"
  pqr NDI Controller/2(TVC_rz) -> Add1/1  "TVC_rz"
  pqr NDI Controller/1("TVC_ry ") -> Add/1  "TVC_ry"
  Add/1 -> TVC_rZ Saturation/1
  Add8/1 -> Rudder Saturation/1
  Add7/1 -> Elevator Saturation/1
  Add6/1 -> Elevator Saturation1/1
  Add5/1 -> Aileron Saturation1/1
  Add4/1 -> Aileron Saturation/1
  Add3/1 -> TVC_lY Saturation/1
  Add1/1 -> TVC_rY Saturation/1
  Add2/1 -> TVC_lZ Saturation/1
  Step/1 -> Switch2/1
  Switch2/1 -> sysID_Onboard_Excitation_System/1(Enable)
  Constant7/1 -> Switch2/3
  Constant8/1 -> Switch2/2
  Manual Switch5/1 -> [cmd_pqr], Sum1/1
  pqr NDI Controller/5(right_aileron) -> Add4/1  "right aileron"
  pqr NDI Controller/6(left_aileron) -> Add5/1  "left aileron"
  pqr NDI Controller/7(right_elevator) -> Add6/1  "right elevator"
  pqr NDI Controller/8(left_elevator) -> Add7/1  "left elevator"
  [NDI_aero_control_M] -> pqr NDI Controller/1(coef M)
  [NDI_aero_control_fast_G] -> pqr NDI Controller/2(control g)
  Mux1/1 -> pqr NDI Controller/3(pqr dot desire)  "pqr dot desire"
  Bus Creator3/1 -> Vehicle/6(LogDataBus)
  [cmd_mu_alpha_beta] -> Bus Creator3/3  "cmd_mu_alpha_beta"
  [cmd_pqr] -> Bus Creator3/4  "cmd_pqr"
  In Bus Element1/1 -> Vehicle/5(EnvData)
  [LEF] -> Bus Creator2/6
  Aerodynamic1/4(LEF) -> [LEF]
  Vehicle/1(PlantData) -> Plant_Data/1, Aerodynamic1/3(AirData), Aerodynamic1/2(PlantData), μαβ NDI Controller/5(PlantData), μαβ NDI Controller/6(AirData), Bus Selector4/1, Rotation Speed(TVC OFF)OK/2(PlantData), Bus Selector1/1, pqr NDI Controller/5(PlantData)
  [DYL] -> Bus Creator3/5  "drag_sideForce_lift"
  cmd_mu/1 -> Mux5/1  "mu command"
  cmd_beta/1 -> Mux5/3  "beta command"
  cmd_alpha/1 -> Mux5/2  "alpha command"
  Constant2/1 -> Bus Creator3/1  "cmd_yz"
  Constant4/1 -> Bus Creator3/2  "cmd_Vt_chi_gamma"

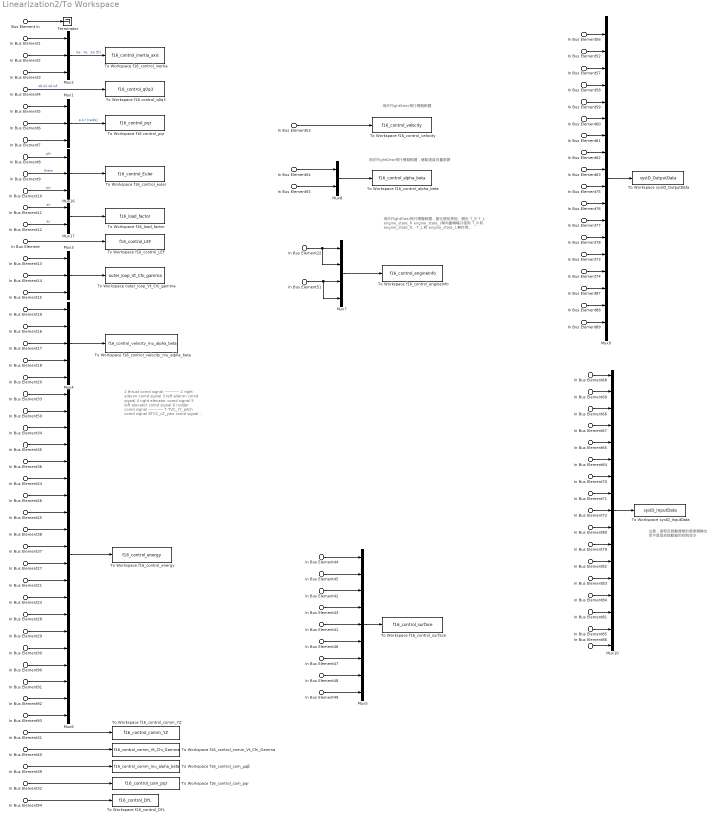
== system Linearization2/To Workspace ==
  note: 1 thrust comd signal
      | -----------
      | 2 right aileron comd signal
      | 3 left aileron comd signal
      | 4 right elevator comd signal
      | 5 left elevator comd signal
      | 6 rudder comd signal
      | -----------
      | 7 TVC_rY_pitch comd signal
      | 8TVC_rZ_yaw comd signal
      | 9 TVC_lY_pitch comd signal
      | 10TVC_lZ_yaw comd signal
      |
      | 11 thrust signal
      | -----------
      | 12 right aileron signal
      | 13 left aileron signal
      | 14 right elevator signal
      | 15 left elevator signal
      | 16 rudder signal
      | -----------
      | 17 TVC_rY_pitch signal
      | 18 TVC_rZ_yaw signal
      | 19 TVC_lY_pitch signal
      | 20 TVC_lZ_yaw signal
  note: 用於FlightGear飛行模擬軟體
  note: 用於FlightGear飛行模擬軟體，繪製速度向量箭頭
  note: 用於FlightGear飛行模擬軟體，變化尾焰長短、顏色
      | T_R
      | T_L
      | engine_state_R
      | engine_state_L
      |
      | 單向量噴嘴只使用 T_R 和 engine_state_R。
      | T_L 和 engine_state_L 無作用。
  note: 注意：是取自致動器號的感測器輸出
      | 而不是取自致動器的控制命令
  In Bus Element1 : Inport  PortName=PlantData  Element=npos
  In Bus Element2 : Inport  PortName=PlantData  Element=epos
  In Bus Element3 : Inport  PortName=PlantData  Element=altitude
  In Bus Element4 : Inport  PortName=PlantData  Element=q0q1q2q3
  In Bus Element5 : Inport  PortName=PlantData  Element=p
  In Bus Element61 : Inport  PortName=PlantData  Element=p
  In Bus Element6 : Inport  PortName=PlantData  Element=q
  In Bus Element62 : Inport  PortName=PlantData  Element=q
  In Bus Element7 : Inport  PortName=PlantData  Element=r
  In Bus Element63 : Inport  PortName=PlantData  Element=r
  In Bus Element8 : Inport  PortName=PlantData  Element=phi
  In Bus Element58 : Inport  PortName=PlantData  Element=phi
  In Bus Element9 : Inport  PortName=PlantData  Element=theta
  In Bus Element59 : Inport  PortName=PlantData  Element=theta
  In Bus Element10 : Inport  PortName=PlantData  Element=psi
  In Bus Element60 : Inport  PortName=PlantData  Element=psi
  In Bus Element11 : Inport  PortName=PlantData  Element=an
  In Bus Element12 : Inport  PortName=PlantData  Element=ay
  In Bus Element : Inport  PortName=PlantData  Element=AeroActBus.LEF_deg
  In Bus Element80 : Inport  PortName=PlantData  Element=AeroActBus.LEF_deg
  In Bus Element30 : Inport  PortName=PlantData  Element=AeroActBus.Rudder_deg
  In Bus Element41 : Inport  PortName=PlantData  Element=AeroActBus.Rudder_deg
  In Bus Element65 : Inport  PortName=PlantData  Element=AeroActBus.Rudder_deg
  In Bus Element21 : Inport  PortName=PlantData  Element=AeroActBus.right Aileron_deg
  In Bus Element42 : Inport  PortName=PlantData  Element=AeroActBus.right Aileron_deg
  In Bus Element66 : Inport  PortName=PlantData  Element=AeroActBus.right Aileron_deg
  In Bus Element23 : Inport  PortName=PlantData  Element=AeroActBus.left Aileron_deg
  In Bus Element43 : Inport  PortName=PlantData  Element=AeroActBus.left Aileron_deg
  In Bus Element67 : Inport  PortName=PlantData  Element=AeroActBus.left Aileron_deg
  In Bus Element28 : Inport  PortName=PlantData  Element=AeroActBus.right Elevator_deg
  In Bus Element44 : Inport  PortName=PlantData  Element=AeroActBus.right Elevator_deg
  In Bus Element68 : Inport  PortName=PlantData  Element=AeroActBus.right Elevator_deg
  In Bus Element29 : Inport  PortName=PlantData  Element=AeroActBus.left Elevator_deg
  In Bus Element45 : Inport  PortName=PlantData  Element=AeroActBus.left Elevator_deg
  In Bus Element69 : Inport  PortName=PlantData  Element=AeroActBus.left Elevator_deg
  In Bus Element79 : Inport  PortName=PlantData  Element=AeroActBus.SB_deg
  In Bus Element{13,19,53,56} (4 alike) : Inport  PortName=PlantData  Element=Vt
  In Bus Element14 : Inport  PortName=PlantData  Element=chi
  In Bus Element88 : Inport  PortName=PlantData  Element=chi
  In Bus Element15 : Inport  PortName=PlantData  Element=gamma
  In Bus Element20 : Inport  PortName=PlantData  Element=gamma
  In Bus Element89 : Inport  PortName=PlantData  Element=gamma
  In Bus Element16 : Inport  PortName=PlantData  Element=alpha
  In Bus Element54 : Inport  PortName=PlantData  Element=alpha
  In Bus Element52 : Inport  PortName=PlantData  Element=alpha
  In Bus Element17 : Inport  PortName=PlantData  Element=beta
  In Bus Element55 : Inport  PortName=PlantData  Element=beta
  In Bus Element57 : Inport  PortName=PlantData  Element=beta
  In Bus Element18 : Inport  PortName=PlantData  Element=mu
  In Bus Element87 : Inport  PortName=PlantData  Element=mu
  In Bus Element33 : Inport  PortName=PlantData  Element=fadec_cmd.thrust
  In Bus Element25 : Inport  PortName=PlantData  Element=fadec_cmd.TVC_rz
  In Bus Element26 : Inport  PortName=PlantData  Element=fadec_cmd.TVC_ry
  In Bus Element37 : Inport  PortName=PlantData  Element=fadec_cmd.TVC_lz
  In Bus Element38 : Inport  PortName=PlantData  Element=fadec_cmd.TVC_ly
  In Bus Element24 : Inport  PortName=PlantData  Element=fcs_cmd.rudder
  In Bus Element34 : Inport  PortName=PlantData  Element=fcs_cmd.left aileron
  In Bus Element35 : Inport  PortName=PlantData  Element=fcs_cmd.right elevator
  In Bus Element36 : Inport  PortName=PlantData  Element=fcs_cmd.left elevator
  In Bus Element50 : Inport  PortName=PlantData  Element=fcs_cmd.right aileron
  In Bus Element27 : Inport  PortName=PlantData  Element=PropBus.T
  In Bus Element22 : Inport  PortName=PlantData  Element=PropBus.T
  In Bus Element51 : Inport  PortName=PlantData  Element=PropBus.engine_state
  In Bus Element82 : Inport  PortName=PlantData  Element=PropBus.Tx
  In Bus Element83 : Inport  PortName=PlantData  Element=PropBus.Ty
  In Bus Element84 : Inport  PortName=PlantData  Element=PropBus.Tz
  In Bus Element73 : Inport  PortName=PlantData  Element=ay_offset
  In Bus Element74 : Inport  PortName=PlantData  Element=az_offset
  In Bus Element75 : Inport  PortName=PlantData  Element=p_dot
  In Bus Element76 : Inport  PortName=PlantData  Element=q_dot
  In Bus Element77 : Inport  PortName=PlantData  Element=r_dot
  In Bus Element85 : Inport  PortName=PlantData  Element=f
  In Bus Element86 : Inport  PortName=PlantData  Element=N
  In Bus Element90 : Inport  PortName=PlantData  Element=PropActBus.TVC_ry_pitch_deg
  In Bus Element46 : Inport  PortName=PlantData  Element=PropActBus.TVC_ry_pitch_deg
  In Bus Element64 : Inport  PortName=PlantData  Element=PropActBus.TVC_ry_pitch_deg
  In Bus Element91 : Inport  PortName=PlantData  Element=PropActBus.TVC_rz_yaw_deg
  In Bus Element47 : Inport  PortName=PlantData  Element=PropActBus.TVC_rz_yaw_deg
  In Bus Element70 : Inport  PortName=PlantData  Element=PropActBus.TVC_rz_yaw_deg
  In Bus Element92 : Inport  PortName=PlantData  Element=PropActBus.TVC_ly_pitch_deg
  In Bus Element48 : Inport  PortName=PlantData  Element=PropActBus.TVC_ly_pitch_deg
  In Bus Element71 : Inport  PortName=PlantData  Element=PropActBus.TVC_ly_pitch_deg
  In Bus Element93 : Inport  PortName=PlantData  Element=PropActBus.TVC_lz_yaw_deg
  In Bus Element49 : Inport  PortName=PlantData  Element=PropActBus.TVC_lz_yaw_deg
  In Bus Element72 : Inport  PortName=PlantData  Element=PropActBus.TVC_lz_yaw_deg
  In Bus Element78 : Inport  PortName=PlantData  Element=ax_offset
  In Bus Element32 : Inport  PortName=PlantData  Element=LogDataBus.cmd_pqr
  In Bus Element39 : Inport  PortName=PlantData  Element=LogDataBus.cmd_mu_alpha_beta
  In Bus Element31 : Inport  PortName=PlantData  Element=LogDataBus.cmd_yz
  In Bus Element40 : Inport  PortName=PlantData  Element=LogDataBus.cmd_Vt_chi_gamma
  In Bus Element94 : Inport  PortName=PlantData  Element=LogDataBus.drag_sideForce_lift
  Bus Element In : Inport  Port=2  PortName=EnvData
  In Bus Element81 : Inport  Port=2  PortName=EnvData  Element=AirDensity
  Mux{1..3,16} (4 alike) : Mux  Inputs=3
  Mux10 : Mux  Inputs=17
  Mux17 : Mux  Inputs=2
  Mux4 : Mux  Inputs=5
  Mux5 : Mux  Inputs=9
  Mux6 : Mux  Inputs=20
  Mux7 : Mux
  Mux8 : Mux  Inputs=2
  Mux9 : Mux  Inputs=18
  Terminator : Terminator
  To Workspace f16 control_pqr : ToWorkspace  VariableName=f16_control_pqr  SaveFormat=Timeseries  SampleTime=-1
  To Workspace f16 control_q0q3 : ToWorkspace  VariableName=f16_control_q0q3  SaveFormat=Timeseries  SampleTime=-1
  To Workspace f16_control_DYL : ToWorkspace  VariableName=f16_control_DYL  SaveFormat=Timeseries  SampleTime=-1
  To Workspace f16_control_LEF : ToWorkspace  VariableName=f16_control_LEF  SaveFormat=Timeseries  SampleTime=-1
  To Workspace f16_control_alpha_beta : ToWorkspace  VariableName=f16_control_alpha_beta  SaveFormat=Timeseries  SampleTime=-1
  To Workspace f16_control_com_pqr : ToWorkspace  VariableName=f16_control_com_pqr  SaveFormat=Timeseries  SampleTime=-1
  To Workspace f16_control_com_μαβ : ToWorkspace  VariableName=f16_control_comm_mu_alpha_beta  SaveFormat=Timeseries  SampleTime=-1
  To Workspace f16_control_comm_Vt_Chi_Gamma : ToWorkspace  VariableName=f16_control_comm_Vt_Chi_Gamma  SaveFormat=Timeseries  SampleTime=-1
  To Workspace f16_control_comm_YZ : ToWorkspace  VariableName=f16_control_comm_YZ  SaveFormat=Timeseries  SampleTime=-1
  To Workspace f16_control_energy : ToWorkspace  VariableName=f16_control_energy  SaveFormat=Timeseries  SampleTime=-1
  To Workspace f16_control_engineInfo : ToWorkspace  VariableName=f16_control_engineInfo  SaveFormat=Timeseries  SampleTime=-1
  To Workspace f16_control_euler : ToWorkspace  VariableName=f16_control_Euler  SaveFormat=Timeseries  SampleTime=-1
  To Workspace f16_control_inertia : ToWorkspace  VariableName=f16_control_inertia_axis  SaveFormat=Timeseries  SampleTime=-1
      settings: Save2DSignal=2-D array (concatenate along first dimension)
  To Workspace f16_control_surface : ToWorkspace  VariableName=f16_control_surface  SaveFormat=Timeseries  SampleTime=-1
  To Workspace f16_control_velocity : ToWorkspace  VariableName=f16_control_velocity  SaveFormat=Timeseries  SampleTime=-1
  To Workspace f16_control_velocity_mu_alpha_beta : ToWorkspace  VariableName=f16_control_velocity_mu_alpha_beta  SaveFormat=Timeseries  SampleTime=-1
  To Workspace f16_load_factor : ToWorkspace  VariableName=f16_load_factor  SaveFormat=Timeseries  SampleTime=-1
  To Workspace outer_loop_Vt_Chi_gamma : ToWorkspace  VariableName=outer_loop_Vt_Chi_gamma  SaveFormat=Timeseries  SampleTime=-1
  To Workspace sysID_InputData : ToWorkspace  VariableName=sysID_InputData  SaveFormat=Timeseries  SampleTime=sysID_DAQ.sampleTime
  To Workspace sysID_OutputData : ToWorkspace  VariableName=sysID_OutputData  SaveFormat=Timeseries  SampleTime=sysID_DAQ.sampleTime
  wires:
  Mux2/1 -> To Workspace f16_control_inertia/1  "Xe   Ye   Ze (ft)"
  Mux16/1 -> To Workspace f16_control_euler/1
  In Bus Element9/1 -> Mux16/2  "theta"
  In Bus Element10/1 -> Mux16/3  "psi"
  In Bus Element4/1 -> To Workspace f16 control_q0q3/1  "q0 q1 q2 q3"
  In Bus Element11/1 -> Mux17/1  "an"
  In Bus Element8/1 -> Mux16/1  "phi"
  Mux17/1 -> To Workspace f16_load_factor/1
  In Bus Element12/1 -> Mux17/2  "ay"
  Mux1/1 -> To Workspace f16 control_pqr/1  "p q r (rad/s)"
  In Bus Element5/1 -> Mux1/1
  In Bus Element6/1 -> Mux1/2
  In Bus Element7/1 -> Mux1/3
  In Bus Element1/1 -> Mux2/1
  In Bus Element2/1 -> Mux2/2
  In Bus Element3/1 -> Mux2/3
  In Bus Element/1 -> To Workspace f16_control_LEF/1
  In Bus Element13/1 -> Mux3/1
  In Bus Element14/1 -> Mux3/2
  In Bus Element15/1 -> Mux3/3
  Mux3/1 -> To Workspace outer_loop_Vt_Chi_gamma/1
  In Bus Element19/1 -> Mux4/1
  In Bus Element16/1 -> Mux4/2
  In Bus Element17/1 -> Mux4/3
  In Bus Element18/1 -> Mux4/4
  In Bus Element20/1 -> Mux4/5
  Mux4/1 -> To Workspace f16_control_velocity_mu_alpha_beta/1
  Mux6/1 -> To Workspace f16_control_energy/1
  Bus Element In/1 -> Terminator/1
  In Bus Element33/1 -> Mux6/1
  In Bus Element50/1 -> Mux6/2
  In Bus Element34/1 -> Mux6/3
  In Bus Element35/1 -> Mux6/4
  In Bus Element36/1 -> Mux6/5
  In Bus Element24/1 -> Mux6/6
  In Bus Element27/1 -> Mux6/11
  In Bus Element21/1 -> Mux6/12
  In Bus Element23/1 -> Mux6/13
  In Bus Element28/1 -> Mux6/14
  In Bus Element29/1 -> Mux6/15
  In Bus Element30/1 -> Mux6/16
  In Bus Element90/1 -> Mux6/17
  In Bus Element91/1 -> Mux6/18
  In Bus Element92/1 -> Mux6/19
  In Bus Element93/1 -> Mux6/20
  In Bus Element41/1 -> Mux5/5
  In Bus Element47/1 -> Mux5/7
  In Bus Element49/1 -> Mux5/9
  In Bus Element48/1 -> Mux5/8
  In Bus Element46/1 -> Mux5/6
  In Bus Element44/1 -> Mux5/1
  In Bus Element45/1 -> Mux5/2
  In Bus Element42/1 -> Mux5/3
  In Bus Element43/1 -> Mux5/4
  Mux5/1 -> To Workspace f16_control_surface/1
  In Bus Element26/1 -> Mux6/7
  In Bus Element25/1 -> Mux6/8
  In Bus Element38/1 -> Mux6/9
  In Bus Element37/1 -> Mux6/10
  Mux8/1 -> To Workspace f16_control_alpha_beta/1
  In Bus Element53/1 -> To Workspace f16_control_velocity/1
  In Bus Element55/1 -> Mux8/2
  In Bus Element54/1 -> Mux8/1
  Mux7/1 -> To Workspace f16_control_engineInfo/1
  In Bus Element22/1 -> Mux7/2, Mux7/1
  In Bus Element51/1 -> Mux7/4, Mux7/3
  In Bus Element78/1 -> Mux9/13
  In Bus Element65/1 -> Mux10/5
  In Bus Element75/1 -> Mux9/10
  In Bus Element80/1 -> Mux10/10
  In Bus Element52/1 -> Mux9/2
  In Bus Element79/1 -> Mux10/11
  In Bus Element59/1 -> Mux9/5
  In Bus Element62/1 -> Mux9/8
  In Bus Element83/1 -> Mux10/13
  In Bus Element73/1 -> Mux9/14
  In Bus Element71/1 -> Mux10/8
  In Bus Element60/1 -> Mux9/6
  In Bus Element61/1 -> Mux9/7
  In Bus Element68/1 -> Mux10/1
  In Bus Element77/1 -> Mux9/12
  In Bus Element66/1 -> Mux10/3
  In Bus Element72/1 -> Mux10/9
  In Bus Element69/1 -> Mux10/2
  In Bus Element70/1 -> Mux10/7
  In Bus Element63/1 -> Mux9/9
  In Bus Element58/1 -> Mux9/4
  In Bus Element57/1 -> Mux9/3
  In Bus Element86/1 -> Mux10/17
  In Bus Element67/1 -> Mux10/4
  In Bus Element88/1 -> Mux9/17
  In Bus Element85/1 -> Mux10/16
  In Bus Element76/1 -> Mux9/11
  In Bus Element84/1 -> Mux10/14
  In Bus Element81/1 -> Mux10/15
  In Bus Element82/1 -> Mux10/12
  In Bus Element87/1 -> Mux9/16
  In Bus Element74/1 -> Mux9/15
  In Bus Element89/1 -> Mux9/18
  In Bus Element64/1 -> Mux10/6
  Mux10/1 -> To Workspace sysID_InputData/1
  In Bus Element56/1 -> Mux9/1
  Mux9/1 -> To Workspace sysID_OutputData/1
  In Bus Element32/1 -> To Workspace f16_control_com_pqr/1
  In Bus Element39/1 -> To Workspace f16_control_com_μαβ/1
  In Bus Element31/1 -> To Workspace f16_control_comm_YZ/1
  In Bus Element40/1 -> To Workspace f16_control_comm_Vt_Chi_Gamma/1
  In Bus Element94/1 -> To Workspace f16_control_DYL/1

== system Linearization2/Environment/Dynamic Pressure ==
  Vt : Inport
  rho : Inport  Port=2
  1/2rhoV^2 : Gain  Gain=1/2  SaturateOnIntegerOverflow=on  OutDataTypeStr=Inherit: Same as input  ParamDataTypeStr=Inherit: Same as input
  Product2 : Product  InputSameDT=on  SaturateOnIntegerOverflow=on  OutDataTypeStr=Inherit: Same as first input
  Square : Math  Operator=square  SignedPower=on
  qbar : Outport
  wires:
  rho/1 -> Product2/2
  Square/1 -> Product2/1
  1/2rhoV^2/1 -> qbar/1
  Product2/1 -> 1/2rhoV^2/1
  Vt/1 -> Square/1

== system Linearization2/Environment/ISP  ==
  note: 1 T
      | 2 a (Speed of sound)
      | 3 P
      | 4 rho
      | 5 g
      | 6 mu (Coefficient of viscosity)
  h(m) : Inport
  Demux : Demux  Outputs=[1,1,1,1,1,1]
      settings: DisplayOption=none
  MATLAB Function : MATLAB Function  TreatAsAtomicUnit=on
  end8 : Terminator
  end9 : Terminator
  T (K) : Outport  VectorParamsAs1DForOutWhenUnconnected=off
  a (m/s) : Outport  Port=2  VectorParamsAs1DForOutWhenUnconnected=off
  P (HPa) : Outport  Port=3  VectorParamsAs1DForOutWhenUnconnected=off
  rho (kg/m^3) : Outport  Port=4  VectorParamsAs1DForOutWhenUnconnected=off
  wires:
  MATLAB Function/1(ISP_output) -> Demux/1
  h(m)/1 -> MATLAB Function/1(h)
  Demux/4 -> rho (kg/m^3)/1  "rho(kg/m^3)"
  Demux/2 -> a (m/s)/1  "a(m/s)"
  Demux/1 -> T (K)/1  "T(K)"
  Demux/5 -> end8/1  "g (m/s^2)"
  Demux/6 -> end9/1  "mu"
  Demux/3 -> P (HPa)/1  "P(Pa)"

== system Linearization2/Environment/Mach Number ==
  Vt : Inport
  a : Inport  Port=2
  Product1 : Product  Inputs=*/  InputSameDT=on  SaturateOnIntegerOverflow=on  OutDataTypeStr=Inherit: Same as first input
  Mach : Outport  Unit=1  VectorParamsAs1DForOutWhenUnconnected=off
  wires:
  Vt/1 -> Product1/1
  a/1 -> Product1/2
  Product1/1 -> Mach/1
